simulink model "untitled1"  (R2024a)
settings: Solver=VariableStepAuto  StartTime=0.0  StopTime=180  RelTol=1e-3
libraries: dspfdesign x10, dspmathops x10, dspsnks4 x1, dspvision x1
settings Model: Creator=Me  LastModifiedBy=Me

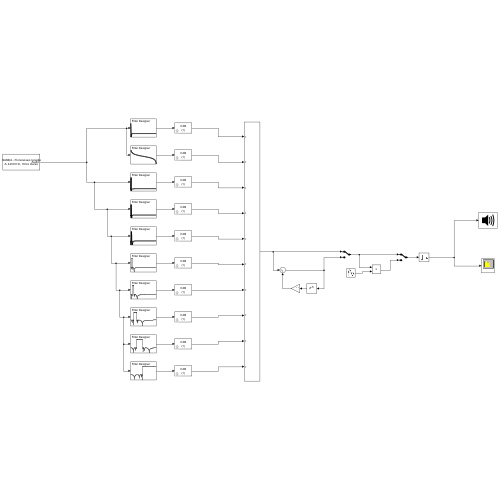
[thumbnail: Simulink's stored preview of the top-level diagram]
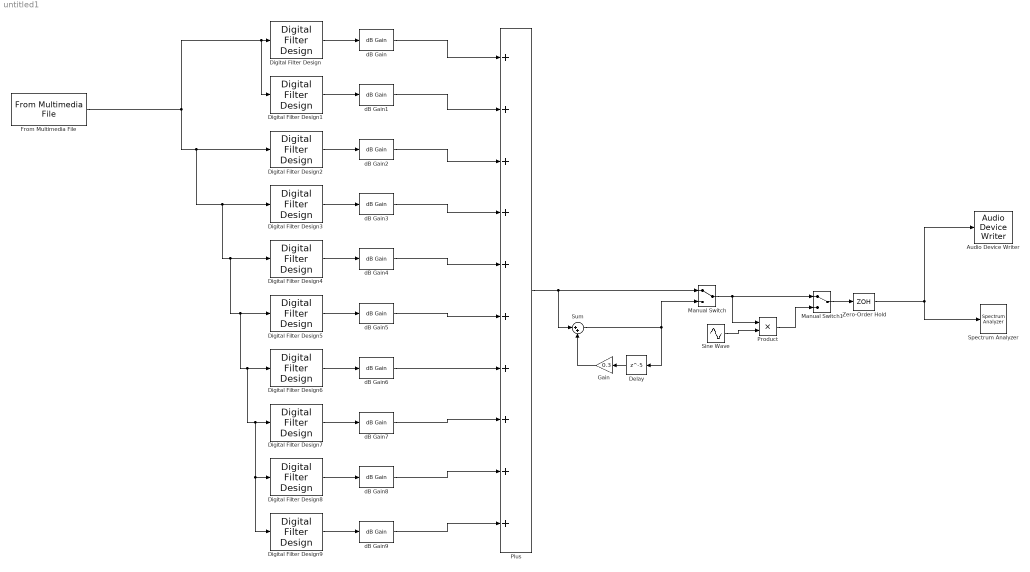
== system untitled1 ==
  Audio Device Writer : dspsnks4/Audio Device Writer  Driver=DirectSound  Device=Default  InheritSampleRate=on  SampleRate=44100  BitDepth=16-bit integer  BufferSize=4096  NumBuffers=10  DefaultOutputChannelMapping=on  OutputChannelMapping=1:2  OutputNumUnderrunSamples=off  DriverIdx=1  DeviceWarnFlag=''
  Delay : Delay  DelayLength=5  InitialCondition=0
  Digital Filter Design{,1..9} (10 alike) : dspfdesign/Digital Filter Design  mwdsp_browser_bugfix_var=off
  From Multimedia File : dspvision/From Multimedia File  inputFilename=C:\Users\Me\Documents\INSTASAMKA - Я отключаю телефон.wav  readRange=[1 Inf]  loop=on  numPlays=inf  outputStreams=Audio only  videoDataType=single  audioDataType=double  inheritSampleTime=on  userDefinedSampleTime=1/30  noAudioOutput=off  isIntensityVideo=off  fourcc=RGB  colorVideoFormat=Separate color signals  outputEOF=off  dataOrg=Column-major  audioFrameSize=1024  computeAudioFrameSize=off  outSamplingMode=Sample based
      settings: LibrarySourceBlock=audiosources/From Multimedia File
  Gain : Gain  Gain=0.3
  Manual Switch : ManualSwitch
  Manual Switch1 : ManualSwitch
  Plus : Sum  Inputs=++++++++++
  Product : Product
  Sine Wave : Sin  Frequency=4  SampleTime=0
  Spectrum Analyzer : SpectrumAnalyzer  WindowPosition=[837.000000,281.000000,800.000000,500.000000,]  ScopeFrameLocation=window  SampleRateSource=Property  SampleRate=44.1e3  PlotAsTwoSidedSpectrum=off  FrequencySpan=Start and stop frequencies  StartFrequency=20  StopFrequency=20e3  YLimits=[-103.68653942,24.75505879]  SelectedToolstripTab=spectrumAnalyzerToolstrip.spectrumTab
  Sum : Sum  Inputs=|++
  Zero-Order Hold : ZeroOrderHold  SampleTime=-1
  dB Gain{,1..9} (10 alike) : dspmathops/dB Gain  dB=0  intype=Amplitude
  wires:
  From Multimedia File/1 -> Digital Filter Design9/1, Digital Filter Design8/1, Digital Filter Design7/1, Digital Filter Design6/1, Digital Filter Design5/1, Digital Filter Design4/1, Digital Filter Design3/1, Digital Filter Design2/1, Digital Filter Design1/1, Digital Filter Design/1
  dB Gain/1 -> Plus/1
  dB Gain1/1 -> Plus/2
  dB Gain2/1 -> Plus/3
  dB Gain3/1 -> Plus/4
  dB Gain4/1 -> Plus/5
  dB Gain5/1 -> Plus/6
  dB Gain6/1 -> Plus/7
  dB Gain7/1 -> Plus/8
  dB Gain8/1 -> Plus/9
  dB Gain9/1 -> Plus/10
  Digital Filter Design/1 -> dB Gain/1
  Digital Filter Design1/1 -> dB Gain1/1
  Digital Filter Design2/1 -> dB Gain2/1
  Digital Filter Design3/1 -> dB Gain3/1
  Digital Filter Design4/1 -> dB Gain4/1
  Digital Filter Design5/1 -> dB Gain5/1
  Digital Filter Design6/1 -> dB Gain6/1
  Digital Filter Design7/1 -> dB Gain7/1
  Digital Filter Design8/1 -> dB Gain8/1
  Digital Filter Design9/1 -> dB Gain9/1
  Plus/1 -> Manual Switch/1, Sum/1
  Sum/1 -> Manual Switch/2, Delay/1
  Delay/1 -> Gain/1
  Gain/1 -> Sum/2
  Manual Switch/1 -> Product/1, Manual Switch1/1
  Product/1 -> Manual Switch1/2
  Manual Switch1/1 -> Zero-Order Hold/1
  Zero-Order Hold/1 -> Spectrum Analyzer/1, Audio Device Writer/1
  Sine Wave/1 -> Product/2
